simulink model "float_re"  (R2025a)
settings: Solver=VariableStepAuto  StartTime=0.0  StopTime=500  RelTol=1e-3
libraries: slpidlib x1
settings Model: Creator=cdcg1  LastModifiedBy=cdcg1

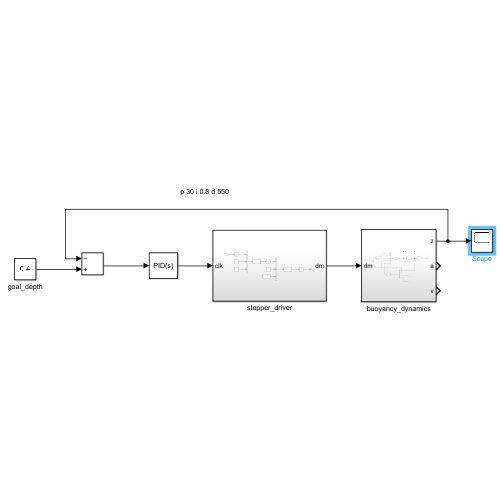
[thumbnail: Simulink's stored preview of the top-level diagram]
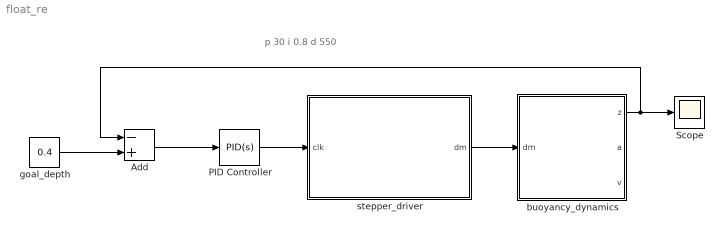
== system float_re ==
  note: p 30 i 0.8 d 550
  Add : Sum  Inputs=-+
  PID Controller : slpidlib/PID Controller  Controller=PID  Form=Parallel  TimeDomain=Continuous-time  UseExternalTs=off  SampleTime=-1  IntegratorMethod=Forward Euler  FilterMethod=Forward Euler  ControllerParametersSource=internal  P=30  I=0.8  UseKiTs=off  D=550  UseExternalDerivativeSource=off  N=100  UseFilter=on  TunerSelectOption=Transfer Function Based (PID Tuner App)  InitialConditionSource=internal  InitialConditionForIntegrator=0  InitialConditionForFilter=0  DifferentiatorICPrevScaledInput=0  ExternalReset=none  TrackingMode=off  Kt=1  LimitOutput=off  SatLimitsSource=internal  UpperSaturationLimit=inf  LowerSaturationLimit=-inf  LinearizeAsGain=on  AntiWindupMode=none  Kb=1  LimitIntegrator=off  UpperIntegratorSaturationLimit=inf  LowerIntegratorSaturationLimit=-inf  POutMin=[]  POutMax=[]  IOutMin=[]  IOutMax=[]  DOutMin=[]  DOutMax=[]  NOutMin=[]  NOutMax=[]  SumOutMin=[]  SumOutMax=[]  SaturationOutMin=[]  SaturationOutMax=[]  PParamMin=[]  PParamMax=[]  IParamMin=[]  IParamMax=[]  DParamMin=[]  DParamMax=[]  NParamMin=[]  NParamMax=[]  KbParamMin=[]  KbParamMax=[]  KtParamMin=[]  KtParamMax=[]  KbOutMin=[]  KbOutMax=[]  KtOutMin=[]  KtOutMax=[]  IntegratorOutMin=[]  IntegratorOutMax=[]  FilterOutMin=[]  FilterOutMax=[]  SumI1OutMin=[]  SumI1OutMax=[]  SumI2OutMin=[]  SumI2OutMax=[]  SumI3OutMin=[]  SumI3OutMax=[]  SumI4OutMin=[]  SumI4OutMax=[]  SumDOutMin=[]  SumDOutMax=[]  DifferentiatorOutMin=[]  DifferentiatorOutMax=[]  FilterDiffOutCoefMin=[]  FilterDiffOutCoefMax=[]  ReciprocalOutMin=[]  ReciprocalOutMax=[]  SumDenOutMin=[]  SumDenOutMax=[]  SumNumOutMin=[]  SumNumOutMax=[]  DivideOutMin=[]  DivideOutMax=[]  UdiffTsProdOutMin=[]  UdiffTsProdOutMax=[]  NTsProdOutMin=[]  NTsProdOutMax=[]  UintegralTsProdOutMin=[]  UintegralTsProdOutMax=[]  UngainTsProdOutMin=[]  UngainTsProdOutMax=[]  ClampingZeroOutDataTypeStr=Inherit: Inherit via back propagation  ClampingZeroOutMin=[]  ClampingZeroOutMax=[]  FilterDenConstantOutDataTypeStr=Inherit: Inherit via back propagation  FilterDenConstantOutMin=[]  FilterDenConstantOutMax=[]  PCopyOutDataTypeStr=Inherit: Inherit via back propagation  PCopyOutMin=[]  PCopyOutMax=[]  NCopyOutDataTypeStr=Inherit: Inherit via back propagation  NCopyOutMin=[]  NCopyOutMax=[]  IntegratorContinuousStateAttributes=''  IntegratorStateMustResolveToSignalObject=off  IntegratorRTWStateStorageClass=Auto  FilterContinuousStateAttributes=''  FilterStateMustResolveToSignalObject=off  FilterRTWStateStorageClass=Auto  ParallelPVariant=InternalParameters  IdealPVariant=Disabled  IVariant=InternalParameters  DVariant=InternalParameters  IntegratorVariant=Continuous  SatVariant=Disabled  AWVariant=Passthrough  PCopyVariant=Disabled  TRVariant=Disabled  FdbkBlocksVariant=Forward  IdealPFdbkVariant=Disabled  SatFdbkVariant=Disabled  DerivativeFilterVariant=ContFilter  NVariant=InternalParameters  NCopyVariant=Disabled  FilterICVariant=InternalICsFilter  IntegratorICVariant=InternalICs  ExternalResetVariant=Disabled  TRSumVariant=Passthrough  SumFdbkVariant=Disabled  SumVariant=Sum_PID  TsampFilterVariant=InternalTs  TsampNgainVariant=Passthrough  TsampIntegralVariant=Disabled_SignalSpec  ExternalSaturationOutDataTypeStr=Inherit: Same as second input  DerivativeSourceVariant=ErrorSignal  PreIntVariant=InternalPreInt
  Scope : Scope
      settings: ActiveDisplayYMinimum=0.16695792765058809  ActiveDisplayYMaximum=0.74417844595099569
  buoyancy_dynamics : Subsystem
  goal_depth : Constant  Value=0.4
  stepper_driver : Subsystem
  wires:
  goal_depth/1 -> Add/2
  buoyancy_dynamics/1(z) -> Scope/1, Add/1
  Add/1 -> PID Controller/1
  PID Controller/1 -> stepper_driver/1(clk)
  stepper_driver/1(dm) -> buoyancy_dynamics/1(dm)

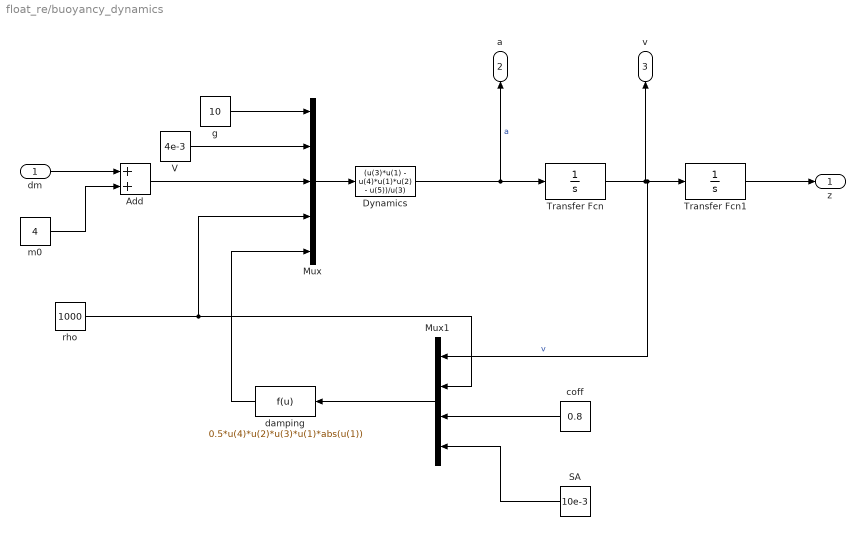
== system float_re/buoyancy_dynamics ==
  dm : Inport
  Add : Sum
  Dynamics : Fcn  Expr=(u(3)*u(1) - u(4)*u(1)*u(2) - u(5))/u(3)
  Mux : Mux  Inputs=5
  Mux1 : Mux
  SA : Constant  Value=10e-3
  Transfer Fcn : TransferFcn  Denominator=[1 0]
  Transfer Fcn1 : TransferFcn  Denominator=[1 0]
  V : Constant  Value=4e-3
  coff : Constant  Value=0.8
  damping : Fcn  Expr=0.5*u(4)*u(2)*u(3)*u(1)*abs(u(1))
  g : Constant  Value=10
  m0 : Constant  Value=4
  rho : Constant  Value=1000
  z : Outport
  a : Outport  Port=2
  v : Outport  Port=3
  wires:
  Add/1 -> Mux/3
  Mux1/1 -> damping/1
  rho/1 -> Mux1/2, Mux/4
  Transfer Fcn/1 -> Transfer Fcn1/1, Mux1/1, v/1  "v"
  SA/1 -> Mux1/4
  Dynamics/1 -> a/1, Transfer Fcn/1  "a"
  Mux/1 -> Dynamics/1
  g/1 -> Mux/1
  m0/1 -> Add/2
  dm/1 -> Add/1
  Transfer Fcn1/1 -> z/1
  V/1 -> Mux/2
  coff/1 -> Mux1/3
  damping/1 -> Mux/5

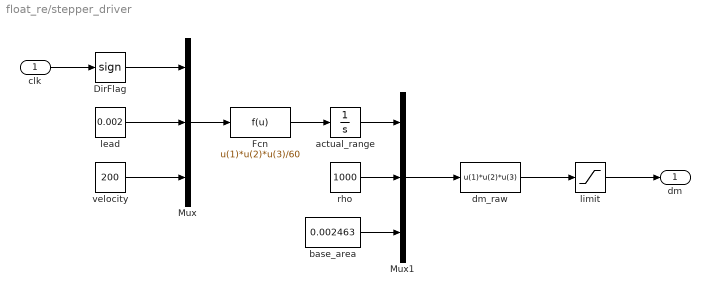
== system float_re/stepper_driver ==
  clk : Inport
  DirFlag : Signum
  Fcn : Fcn  Expr=u(1)*u(2)*u(3)/60
  Mux : Mux  Inputs=3
  Mux1 : Mux  Inputs=3
  actual_range : Integrator
  base_area : Constant  Value=0.002463
  dm_raw : Fcn  Expr=u(1)*u(2)*u(3)
  lead : Constant  Value=0.002
  limit : Saturate  UpperLimit=0.15  LowerLimit=-0.15
  rho : Constant  Value=1000
  velocity : Constant  Value=200
  dm : Outport
  wires:
  lead/1 -> Mux/2
  Mux/1 -> Fcn/1
  clk/1 -> DirFlag/1
  velocity/1 -> Mux/3
  DirFlag/1 -> Mux/1
  Fcn/1 -> actual_range/1
  actual_range/1 -> Mux1/1
  Mux1/1 -> dm_raw/1
  dm_raw/1 -> limit/1
  base_area/1 -> Mux1/3
  rho/1 -> Mux1/2
  limit/1 -> dm/1
